simulink model "Efficiency_Map_ID_Validation_Sim"  (R2019a)
settings: Solver=VariableStepAuto  StartTime=0.0  StopTime=10.0  RelTol=1e-3
undefined symbols (not defined in the file or in its folder): motor_speed, motor_torque, p00, p01, p02, p03, p10, p11, p12, p20, p21, p30
settings Model: Creator=Robert Wygant  LastModifiedBy=hangking
settings DataIOCC: ReturnWorkspaceOutputs=off
settings DebuggingCC: ArithmeticOperatorsInVariantConditions=warning
settings SFSimCC: SimUseLocalCustomCode=off
settings RTWCC: RTWUseLocalCustomCode=off

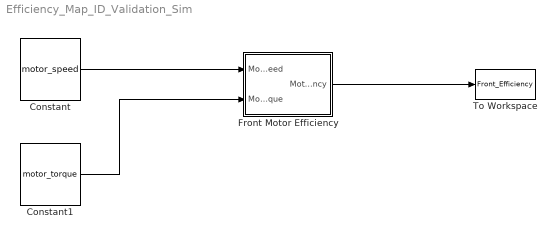
== system Efficiency_Map_ID_Validation_Sim ==
  Constant : Constant  Value=motor_speed
  Constant1 : Constant  Value=motor_torque
  Front Motor Efficiency : Subsystem
      mask Display:
      | color('green')
      | disp("Motor Efficiency")
  To Workspace : ToWorkspace  VariableName=Front_Efficiency  SampleTime=-1
      settings: MaxDataPoints=1  Save2DSignal=2-D array (concatenate along first dimension)
  wires:
  Constant/1 -> Front Motor Efficiency/1(Motor_speed)
  Constant1/1 -> Front Motor Efficiency/2(Motor_torque)
  Front Motor Efficiency/1(Motor_efficiency) -> To Workspace/1

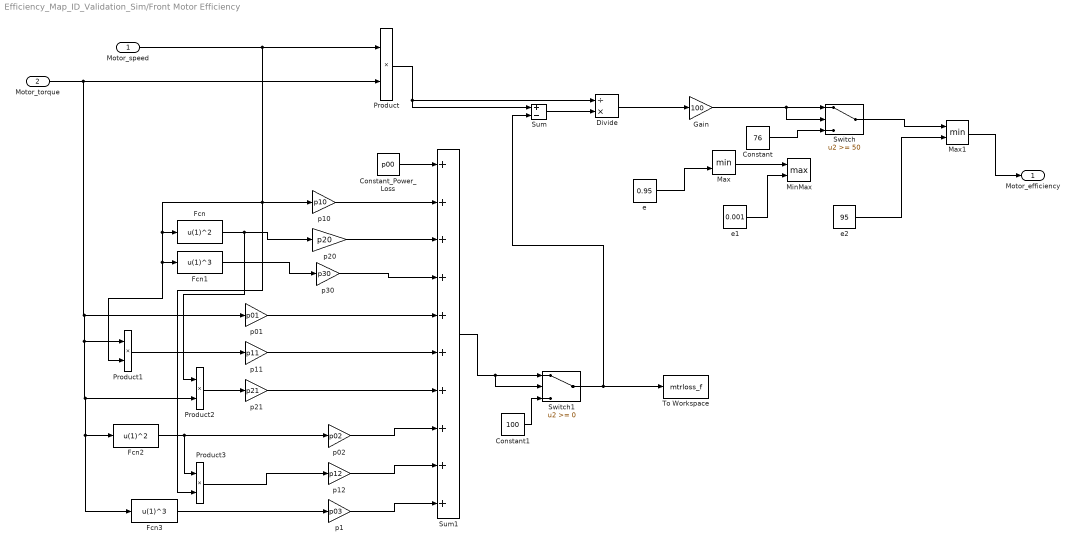
== system Efficiency_Map_ID_Validation_Sim/Front Motor Efficiency ==
  Motor_speed : Inport
  Motor_torque : Inport  Port=2
  Constant : Constant  Value=76
  Constant1 : Constant  Value=100
  Constant_Power_Loss : Constant  Value=p00
  Divide : Product  Inputs=/*
  Fcn : Fcn  Expr=u(1)^2
  Fcn1 : Fcn  Expr=u(1)^3
  Fcn2 : Fcn  Expr=u(1)^2
  Fcn3 : Fcn  Expr=u(1)^3
  Gain : Gain  Gain=100
  Max : MinMax  Inputs=2
  Max1 : MinMax  Inputs=2
  MinMax : MinMax  Function=max  Inputs=2
  Product{,1..3} (4 alike) : Product
  Sum : Sum  Inputs=+-
  Sum1 : Sum  Inputs=++++++++++
  Switch : Switch  Threshold=50
  Switch1 : Switch
  To Workspace : ToWorkspace  VariableName=mtrloss_f  SampleTime=-1
      settings: MaxDataPoints=1  Save2DSignal=2-D array (concatenate along first dimension)
  e : Constant  Value=0.95
  e1 : Constant  Value=0.001
  e2 : Constant  Value=95
  p01 : Gain  Gain=p01
  p02 : Gain  Gain=p02
  p1 : Gain  Gain=p03
  p10 : Gain  Gain=p10
  p11 : Gain  Gain=p11
  p12 : Gain  Gain=p12
  p20 : Gain  Gain=p20
  p21 : Gain  Gain=p21
  p30 : Gain  Gain=p30
  Motor_efficiency : Outport
  wires:
  Max/1 -> MinMax/1
  e/1 -> Max/2
  Fcn3/1 -> p1/1
  p1/1 -> Sum1/10
  p12/1 -> Sum1/9
  Product3/1 -> p12/1
  Motor_torque/1 -> Product/2, p01/1, Product1/1, Product2/2, Fcn2/1, Fcn3/1
  p01/1 -> Sum1/5
  p11/1 -> Sum1/6
  p21/1 -> Sum1/7
  p02/1 -> Sum1/8
  Fcn2/1 -> p02/1, Product3/1
  Product2/1 -> p21/1
  Product1/1 -> p11/1
  p30/1 -> Sum1/4
  Fcn1/1 -> p30/1
  Fcn/1 -> p20/1, Product2/1
  p20/1 -> Sum1/3
  p10/1 -> Sum1/2
  Constant_Power_Loss/1 -> Sum1/1
  Motor_speed/1 -> Product/1, p10/1, Fcn/1, Fcn1/1, Product1/2, Product3/2
  Sum1/1 -> Switch1/2, Switch1/1
  Sum/1 -> Divide/2
  Product/1 -> Divide/1, Sum/1
  e1/1 -> MinMax/2
  Constant1/1 -> Switch1/3
  Switch1/1 -> Sum/2, To Workspace/1
  Divide/1 -> Gain/1
  Constant/1 -> Switch/3
  Gain/1 -> Switch/1, Switch/2
  Switch/1 -> Max1/1
  e2/1 -> Max1/2
  Max1/1 -> Motor_efficiency/1
